simulink model "CompVG_TestBed1_org"  (Simulink 10.0)
settings: Solver=FixedStepDiscrete  StartTime=0.0  StopTime=1  FixedStep=1  RelTol=1e-3  EnableMultiTasking=on
undefined symbols (not defined in the file): MWS, stripchar_TMATS
libraries: Lib_Turbo_CompressorVG_TMATS x1
settings Model: Creator=jwchapm2  LastModifiedBy=annonymous
settings DataIOCC: LimitDataPoints=on
settings OptimizationCC: ExpressionDepthLimit=2147483647
settings DebuggingCC: SolverPrmCheckMsg=warning  StateNameClashWarn=warning
settings GRTTargetCC: GeneratePreprocessorConditionals=Disable all  CombineOutputUpdateFcns=on  GRTInterface=off
settings ConfigComp: CovExternalEMLEnable=off

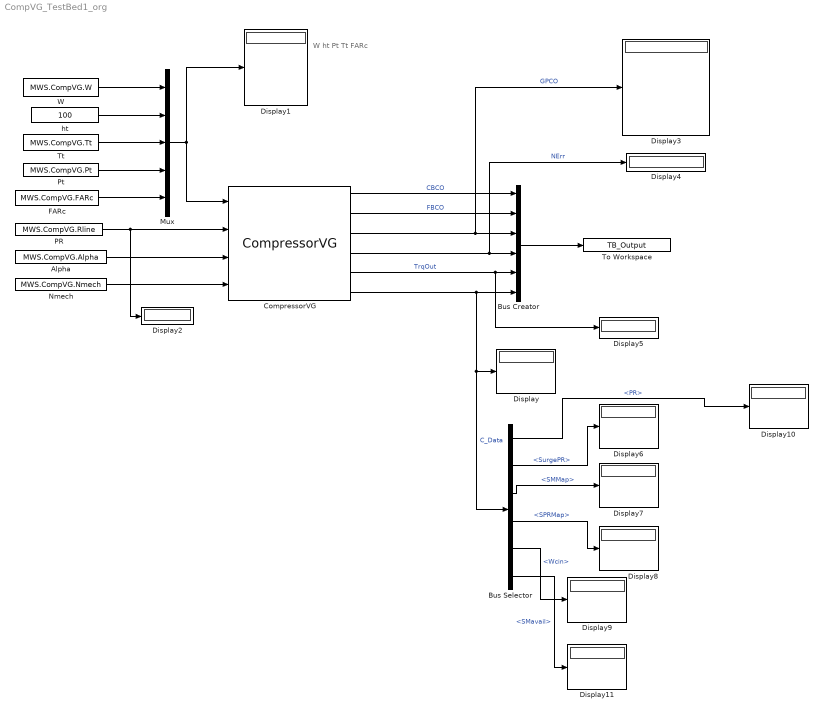
== system CompVG_TestBed1_org ==
  note: W
      | ht
      | Pt
      | Tt
      | FARc
  Alpha : Constant  Value=MWS.CompVG.Alpha
  Bus Selector : BusSelector  OutputSignals=PR,SurgePR,SMMap,SPRMap,Wcin,SMavail
  Bus Creator : BusCreator  Inputs=6
  CompressorVG : Lib_Turbo_CompressorVG_TMATS/CompressorVG  X_C_RlineVec_M=MWS.CompVG.RlineVec  Z_C_AlphaVec_M=MWS.CompVG.AlphaVec  Y_C_Map_NcVec_M=MWS.CompVG.NcVec  T_C_Map_WcArray_M=MWS.CompVG.WcArray  T_C_Map_PRArray_M=MWS.CompVG.PRArray  T_C_Map_EffArray_M=MWS.CompVG.EffArray  s_C_Nc_M=MWS.CompVG.s_Nc  s_C_Wc_M=MWS.CompVG.s_Wc  s_C_PR_M=MWS.CompVG.s_PR  s_C_Eff_M=MWS.CompVG.s_eff  SL_M=off  Scale_M=none  CBLDEN_M=on  C_CBD_M=MWS.CompVG.CBD  C_CBFht_M=MWS.CompVG.CBFht  C_CBFPt_M=MWS.CompVG.CBFPt  FBLDEN_M=on  C_FBD_M=MWS.CompVG.FBD  C_BFht_M=MWS.CompVG.FBht  C_BFPt_M=MWS.CompVG.FBPt  DefSMEn_M=off  SRline_M=1  X_C_Map_WcSurgeVec_M=MWS.CompVG.WcSurgeVec  T_C_Map_PRSurgeVec_M=MWS.CompVG.PRSugeVec  iDesign_M=2  NcDes_M=10000  EffDes_M=0.95  PRDes_M=20  RlineDes_M=2  FVar_M=strcat('iDes_',stripchar_TMATS(gcb),'.bin')  BlkNm_M=double(gcb)  HP_M=off
  Display{,1..11} (12 alike) : Display
  FARc : Constant  Value=MWS.CompVG.FARc
  Mux : Mux  Inputs=5
  Nmech : Constant  Value=MWS.CompVG.Nmech
  PR : Constant  Value=MWS.CompVG.Rline
  Pt : Constant  Value=MWS.CompVG.Pt
  To Workspace : ToWorkspace  VariableName=TB_Output  SampleTime=-1
  Tt : Constant  Value=MWS.CompVG.Tt
  W : Constant  Value=MWS.CompVG.W
  ht : Constant  Value=100
  wires:
  PR/1 -> Display2/1, CompressorVG/2
  W/1 -> Mux/1
  FARc/1 -> Mux/5
  Tt/1 -> Mux/3
  Pt/1 -> Mux/4
  Mux/1 -> CompressorVG/1, Display1/1
  CompressorVG/3 -> Display3/1, Bus Creator/3  "GPCO"
  CompressorVG/4 -> Display4/1, Bus Creator/4  "NErr"
  CompressorVG/5 -> Bus Creator/5, Display5/1  "TrqOut"
  CompressorVG/6 -> Bus Creator/6, Bus Selector/1, Display/1  "C_Data"
  Bus Creator/1 -> To Workspace/1
  ht/1 -> Mux/2
  Nmech/1 -> CompressorVG/4
  CompressorVG/2 -> Bus Creator/2  "FBCO"
  CompressorVG/1 -> Bus Creator/1  "CBCO"
  Alpha/1 -> CompressorVG/3
  Bus Selector/2 -> Display6/1  "<SurgePR>"
  Bus Selector/3 -> Display7/1  "<SMMap>"
  Bus Selector/4 -> Display8/1  "<SPRMap>"
  Bus Selector/5 -> Display9/1  "<Wcin>"
  Bus Selector/1 -> Display10/1  "<PR>"
  Bus Selector/6 -> Display11/1  "<SMavail>"
